simulink model "simnewaveinvertermodel2"  (R2017b)
settings: Solver=VariableStepAuto  StartTime=0.0  StopTime=1  MaxStep=1e-4  RelTol=1e-3
libraries: powerlib x15, powerlib_meascontrol x1
settings Model: Creator=RICHARD MARTIN  LastModifiedBy=RICHARD MARTIN
settings SolverCC: ZeroCrossAlgorithm=Adaptive
settings DebuggingCC: MaxConsecutiveZCsMsg=none

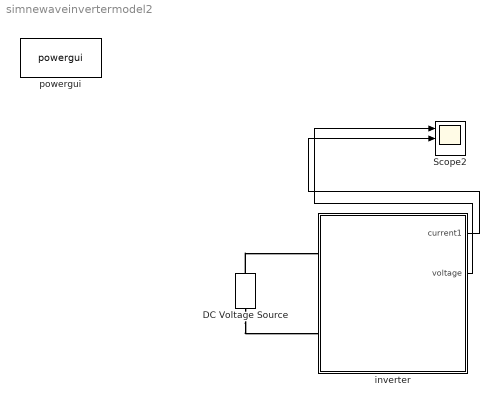
== system simnewaveinvertermodel2 ==
  DC Voltage Source : powerlib/Electrical Sources/DC Voltage Source  Amplitude=100  Measurements=None
  Scope2 : Scope  NumInputPorts=3
  inverter : Subsystem
  powergui : powerlib/powergui  Priority=1  SimulationMode=Continuous  SampleTime=50e-6  frequency=60  Iterations=50  frequencyindice=0  Pbase=100e6  ErrMax=1e-4  UnitsV=kV  UnitsW=MW  buscounter=0  FunctionMessages=off  echomessages=off  EnableUseOfTLC=off  CurrentSourceSwitches=off  DisableSnubberDevices=off  DisableRonSwitches=off  DisableVfSwitches=off  DisplayEquations=off  SolverType=Tustin/Backward Euler (TBE)  Interpol=off  ExternalGateDelay=off  methode=off  Ts=100  x0status=blocks  SPID=on  SwTol=0  HookPort=off  RestoreLinks=warning  ResistiveCurrentMeasurement=off  Frange=[0:2:500]  Ylog=off  Xlog=on  ShowGrid=off  save=off  variable=ZData  structure=0  ZoomFFT=off  StartTime=0.0  cycles=1  DisplayStyle=1  fundamental=60  FreqAxis=off  MaxFrequency=1000  frequencyindicesteady=1  RmsSteady=1  display=off
  wires:
  inverter/1(current1) -> Scope2/2
  inverter/2(voltage) -> Scope2/1
  connections:
  DC Voltage Source/LConn1 -- inverter/LConn2
  DC Voltage Source/RConn1 -- inverter/LConn1

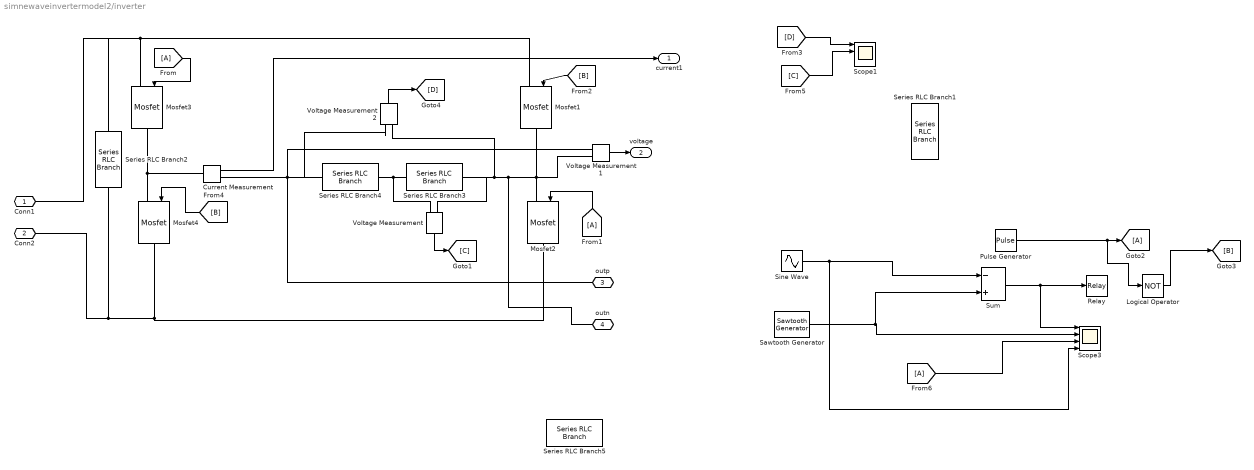
== system simnewaveinvertermodel2/inverter ==
  Current Measurement : powerlib/Measurements/Current Measurement  PhasorSimulation=off  OutputType=Complex  PSBequivalent=0
  Logical Operator : Logic  Operator=NOT  AllPortsSameDT=off  OutDataTypeStr=boolean
  Mosfet{1..4} (4 alike) : powerlib/Power Electronics/Mosfet  Ron=0.1  Lon=0  Rd=0.01  Vfd=0  IC=0  Rs=1e5  Cs=inf  Measurements=off
  Pulse Generator : DiscretePulseGenerator  PulseType=Time based  Period=.02  PulseWidth=50
  Relay : Relay
  Sawtooth Generator : powerlib_meascontrol/Pulse & Signal Generators/Sawtooth Generator  Freq=25e3  Phase=0  Ts=0
      settings: SourceProductName=Simscape Power Systems
  Scope1 : Scope  NumInputPorts=4
  Scope3 : Scope  NumInputPorts=4
  Series RLC Branch1 : powerlib/Elements/Series RLC Branch  LConnTagsString=__new0  RConnTagsString=__new0  BranchType=C  Resistance=100  Inductance=1e-3  SetiL0=off  InitialCurrent=0  Capacitance=4e-3  Setx0=off  InitialVoltage=0  Measurements=None
  Series RLC Branch2 : powerlib/Elements/Series RLC Branch  LConnTagsString=__new0  RConnTagsString=__new0  BranchType=RC  Resistance=1  Inductance=1e-3  SetiL0=off  InitialCurrent=0  Capacitance=1e-6  Setx0=off  InitialVoltage=0  Measurements=None
  Series RLC Branch3 : powerlib/Elements/Series RLC Branch  LConnTagsString=__new0  RConnTagsString=__new0  BranchType=R  Resistance=100  Inductance=30e-6  SetiL0=off  InitialCurrent=0  Capacitance=1e-6  Setx0=off  InitialVoltage=0  Measurements=None
  Series RLC Branch4 : powerlib/Elements/Series RLC Branch  LConnTagsString=__new0  RConnTagsString=__new0  BranchType=L  Resistance=100  Inductance=1  SetiL0=off  InitialCurrent=0  Capacitance=1e-6  Setx0=off  InitialVoltage=0  Measurements=None
  Series RLC Branch5 : powerlib/Elements/Series RLC Branch  LConnTagsString=__new0  RConnTagsString=__new0  BranchType=C  Resistance=100  Inductance=350e-3  SetiL0=off  InitialCurrent=0  Capacitance=10e-6  Setx0=off  InitialVoltage=0  Measurements=None
  Sine Wave : Sin  Amplitude=2  Frequency=2*pi*50  SampleTime=0
  Sum : Sum  Inputs=-+
  Voltage Measurement : powerlib/Measurements/Voltage Measurement  PhasorSimulation=off  OutputType=Complex  PSBequivalent=0
  Voltage Measurement1 : powerlib/Measurements/Voltage Measurement  PhasorSimulation=off  OutputType=Complex  PSBequivalent=0
  Voltage Measurement2 : powerlib/Measurements/Voltage Measurement  PhasorSimulation=off  OutputType=Complex  PSBequivalent=0
  Conn1 : PMIOPort  Port=1  Side=Left
  Conn2 : PMIOPort  Port=2  Side=Left
  outp : PMIOPort  Port=3  Side=Right
  outn : PMIOPort  Port=4  Side=Right
  current1 : Outport
  voltage : Outport  Port=2
  wires:
  Voltage Measurement1/1 -> voltage/1
  Current Measurement/1 -> current1/1
  [A] -> Mosfet2/1
  [A] -> Mosfet3/1
  Sum/1 -> Scope3/1, Relay/1
  Sine Wave/1 -> Sum/1, Scope3/4
  Sawtooth Generator/1 -> Sum/2, Scope3/2
  Logical Operator/1 -> [B]
  [B] -> Mosfet1/1
  [B] -> Mosfet4/1
  Voltage Measurement/1 -> [C]
  Voltage Measurement2/1 -> [D]
  [D] -> Scope1/1
  [C] -> Scope1/2
  [A] -> Scope3/3
  Pulse Generator/1 -> Logical Operator/1, [A]
  connections:
  Mosfet2/RConn1 -- Mosfet4/RConn1 -- Series RLC Branch2/RConn1 -- Conn2/RConn1
  Series RLC Branch3/RConn1 -- Voltage Measurement/LConn2 -- Voltage Measurement2/LConn2 -- outn/RConn1 -- Mosfet2/LConn1 -- Voltage Measurement1/LConn2 -- Mosfet1/RConn1
  Current Measurement/LConn1 -- Mosfet4/LConn1 -- Mosfet3/RConn1
  Voltage Measurement1/LConn1 -- Voltage Measurement2/LConn1 -- Series RLC Branch4/LConn1 -- outp/RConn1 -- Current Measurement/RConn1
  Mosfet1/LConn1 -- Series RLC Branch2/LConn1 -- Conn1/RConn1 -- Mosfet3/LConn1
  Series RLC Branch4/RConn1 -- Series RLC Branch3/LConn1 -- Voltage Measurement/LConn1
